simulink model "BO_Linear"  (R2024b)
settings: Solver=VariableStepAuto  StartTime=0.0  StopTime=10.0  RelTol=1e-3
values from neighbouring files (symbols this model uses):
  plant_ss = plant_ss_q1    [Copy_of_main_final.m]    (also in syst_repr_generator.m = ss(A,B,C,D))
  q20 = 10    [Copy_of_main_final.m]
settings Model: Creator=dsagn  LastModifiedBy=dsagn

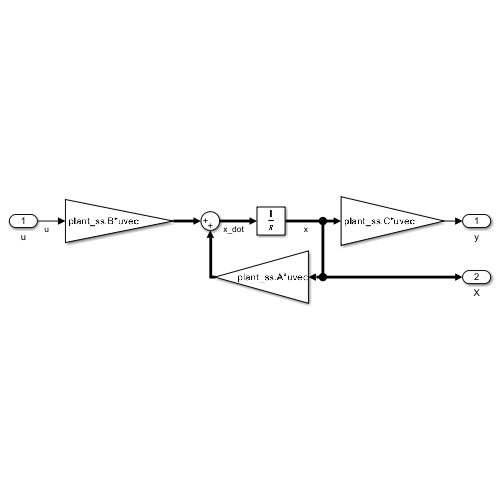
[thumbnail: Simulink's stored preview of the top-level diagram]
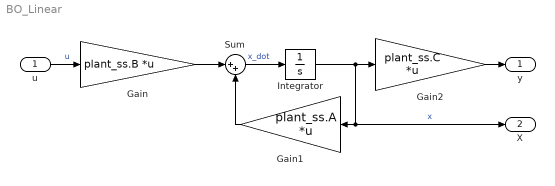
== system BO_Linear ==
  u : Inport
  Gain : Gain  Gain=plant_ss.B  Multiplication=Matrix(K*u) (u vector)
  Gain1 : Gain  Gain=plant_ss.A  Multiplication=Matrix(K*u) (u vector)
  Gain2 : Gain  Gain=plant_ss.C  Multiplication=Matrix(K*u) (u vector)
  Integrator : Integrator  InitialCondition=[0,q20,0,0]
  Sum : Sum  Inputs=|++
  y : Outport  VectorParamsAs1DForOutWhenUnconnected=off
  X : Outport  Port=2
  wires:
  Gain/1 -> Sum/1
  Integrator/1 -> Gain2/1, X/1, Gain1/1  "x"
  Gain1/1 -> Sum/2
  u/1 -> Gain/1  "u"
  Sum/1 -> Integrator/1  "x_dot"
  Gain2/1 -> y/1
